simulink model "proceso_simulacion_1"  (Simulink 7.5)
settings: Solver=ode3  StartTime=0.0  StopTime=16000  FixedStep=0.5  RelTol=1e-3
libraries: realtime_pacer_lib x1
settings Model: Creator=cliente  LastModifiedBy=Administrador

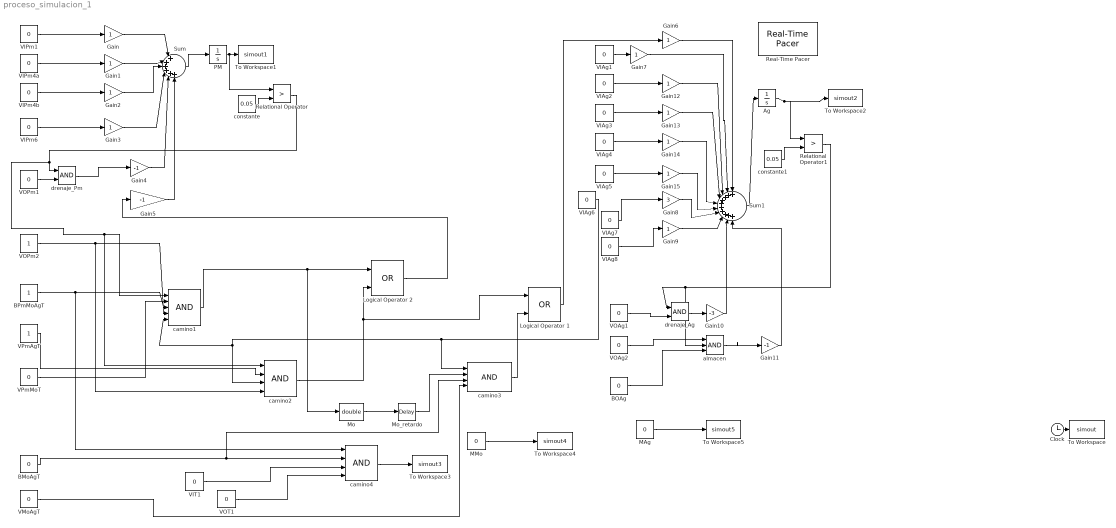
== system proceso_simulacion_1 ==
  Ag : Integrator
  BMoAgT : Constant  Value=0  OutDataType=fixdt(1, 16)  OutScaling=2^0
  BOAg : Constant  Value=0  OutDataType=fixdt(1, 16)  OutScaling=2^0
  BPmMoAgT : Constant  OutDataType=fixdt(1, 16)  OutScaling=2^0
  Clock : Clock
      settings: Decimation=10
  Gain{,1..3,6..7,9,12..15} (11 alike) : Gain  ParameterDataType=fixdt(1, 16)  ParameterScaling=2^0  OutDataType=fixdt(1, 16)  OutScaling=2^0
  Gain10 : Gain  Gain=-3  ParameterDataType=fixdt(1, 16)  ParameterScaling=2^0  OutDataType=fixdt(1, 16)  OutScaling=2^0
  Gain11 : Gain  Gain=-1  ParameterDataType=fixdt(1, 16)  ParameterScaling=2^0  OutDataType=fixdt(1, 16)  OutScaling=2^0
  Gain4 : Gain  Gain=-1  ParameterDataType=fixdt(1, 16)  ParameterScaling=2^0  OutDataType=fixdt(1, 16)  OutScaling=2^0
  Gain5 : Gain  Gain=-1  ParameterDataType=fixdt(1, 16)  ParameterScaling=2^0  OutDataType=fixdt(1, 16)  OutScaling=2^0
  Gain8 : Gain  Gain=3  ParameterDataType=fixdt(1, 16)  ParameterScaling=2^0  OutDataType=fixdt(1, 16)  OutScaling=2^0
  Logical Operator 1 : Logic  Operator=OR  AllPortsSameDT=off  OutDataTypeMode=Specify via dialog  LogicDataType=fixdt(1,16)  OutDataTypeStr=fixdt(1,16)
  Logical Operator 2 : Logic  Operator=OR  AllPortsSameDT=off  OutDataTypeMode=Specify via dialog  LogicDataType=fixdt(1,16)  OutDataTypeStr=fixdt(1,16)
  MAg : Constant  Value=0  OutDataType=fixdt(1, 16)  OutScaling=2^0
  MMo : Constant  Value=0  OutDataType=fixdt(1, 16)  OutScaling=2^0
  Mo : DataTypeConversion  OutDataTypeMode=double  OutDataType=fixdt(1, 16)  OutScaling=2^0  OutDataTypeStr=double
  Mo_retardo : TransportDelay  DelayTime=0.5
  PM : Integrator
  Real-Time Pacer : realtime_pacer_lib/Real-Time Pacer  simTimePerRealTime=1.35
  Relational Operator : RelationalOperator  Operator=>  LogicOutDataTypeMode=boolean  LogicDataType=fixdt(0, 8)  OutDataTypeStr=boolean
  Relational Operator1 : RelationalOperator  Operator=>  LogicOutDataTypeMode=boolean  LogicDataType=fixdt(0, 8)  OutDataTypeStr=boolean
  Sum : Sum  Inputs=|++++++  OutDataType=fixdt(1, 16)  OutScaling=2^0
  Sum1 : Sum  Inputs=++++++++++  OutDataType=fixdt(1, 16)  OutScaling=2^0
  To Workspace : ToWorkspace  VariableName=simout  SampleTime=-1  SaveFormat=Array
  To Workspace1 : ToWorkspace  VariableName=simout1  SampleTime=-1  SaveFormat=Array
  To Workspace2 : ToWorkspace  VariableName=simout2  SampleTime=-1  SaveFormat=Array
  To Workspace3 : ToWorkspace  VariableName=simout3  SampleTime=-1  SaveFormat=Array
  To Workspace4 : ToWorkspace  VariableName=simout4  SampleTime=-1  SaveFormat=Array
  To Workspace5 : ToWorkspace  VariableName=simout5  SampleTime=-1  SaveFormat=Array
  VIAg{1..8} (8 alike) : Constant  Value=0  OutDataType=fixdt(1, 16)  OutScaling=2^0
  VIPm1 : Constant  Value=0  OutDataType=fixdt(1, 16)  OutScaling=2^0
  VIPm4a : Constant  Value=0  OutDataType=fixdt(1, 16)  OutScaling=2^0
  VIPm4b : Constant  Value=0  OutDataType=fixdt(1, 16)  OutScaling=2^0
  VIPm6 : Constant  Value=0  OutDataType=fixdt(1, 16)  OutScaling=2^0
  VIT1 : Constant  Value=0  OutDataType=fixdt(1, 16)  OutScaling=2^0
  VMoAgT : Constant  Value=0  OutDataType=fixdt(1, 16)  OutScaling=2^0
  VOAg1 : Constant  Value=0  OutDataType=fixdt(1, 16)  OutScaling=2^0
  VOAg2 : Constant  Value=0  OutDataType=fixdt(1, 16)  OutScaling=2^0
  VOPm1 : Constant  Value=0  OutDataType=fixdt(1, 16)  OutScaling=2^0
  VOPm2 : Constant  OutDataType=fixdt(1, 16)  OutScaling=2^0
  VOT1 : Constant  Value=0  OutDataType=fixdt(1, 16)  OutScaling=2^0
  VPmAgT : Constant  OutDataType=fixdt(1, 16)  OutScaling=2^0
  VPmMoT : Constant  Value=0  OutDataType=fixdt(1, 16)  OutScaling=2^0
  almacen : Logic  Inputs=3  AllPortsSameDT=off  OutDataTypeMode=Specify via dialog  LogicDataType=fixdt(1,16)  OutDataTypeStr=fixdt(1,16)
  camino1 : Logic  Inputs=5  AllPortsSameDT=off  OutDataTypeMode=Specify via dialog  LogicDataType=fixdt(1,16)  OutDataTypeStr=fixdt(1,16)
  camino2 : Logic  Inputs=4  AllPortsSameDT=off  OutDataTypeMode=Specify via dialog  LogicDataType=fixdt(1,16)  OutDataTypeStr=fixdt(1,16)
  camino3 : Logic  Inputs=4  AllPortsSameDT=off  OutDataTypeMode=boolean  LogicDataType=fixdt(0, 8)  OutDataTypeStr=boolean
  camino4 : Logic  Inputs=4  AllPortsSameDT=off  OutDataTypeMode=Specify via dialog  LogicDataType=fixdt(1,16)  OutDataTypeStr=fixdt(1,16)
  constante : Constant  Value=0.05  OutDataType=fixdt(1, 16)  OutScaling=2^0
  constante1 : Constant  Value=0.05  OutDataType=fixdt(1, 16)  OutScaling=2^0
  drenaje_Ag : Logic  AllPortsSameDT=off  OutDataTypeMode=Specify via dialog  LogicDataType=fixdt(1,16)  OutDataTypeStr=fixdt(1,16)
  drenaje_Pm : Logic  AllPortsSameDT=off  OutDataTypeMode=Specify via dialog  LogicDataType=fixdt(1,16)  OutDataTypeStr=fixdt(1,16)
  wires:
  Gain/1 -> Sum/1
  Gain1/1 -> Sum/2
  Gain2/1 -> Sum/3
  VIPm4b/1 -> Gain2/1
  VIPm4a/1 -> Gain1/1
  VIPm1/1 -> Gain/1
  Sum/1 -> PM/1
  VIPm6/1 -> Gain3/1
  Gain3/1 -> Sum/4
  Gain4/1 -> Sum/5
  Gain5/1 -> Sum/6
  PM/1 -> To Workspace1/1, Relational Operator/1
  Clock/1 -> To Workspace/1
  constante/1 -> Relational Operator/2
  Relational Operator/1 -> drenaje_Pm/1, camino1/1, camino2/1
  VOPm1/1 -> drenaje_Pm/2
  drenaje_Pm/1 -> Gain4/1
  VPmMoT/1 -> camino1/2
  VMoAgT/1 -> camino3/4
  BPmMoAgT/1 -> camino4/1, camino1/3
  BMoAgT/1 -> camino4/2, camino3/3
  camino1/1 -> Logical Operator 2/1, Mo/1
  camino2/1 -> Logical Operator 2/2, Logical Operator 1/1
  Logical Operator 2/1 -> Gain5/1
  VIAg1/1 -> Gain7/1
  VIAg7/1 -> Gain8/1
  VIAg8/1 -> Gain9/1
  Gain6/1 -> Sum1/1
  Gain7/1 -> Sum1/2
  Sum1/1 -> Ag/1
  constante1/1 -> Relational Operator1/2
  Relational Operator1/1 -> drenaje_Ag/1, almacen/2
  VOAg1/1 -> drenaje_Ag/2
  drenaje_Ag/1 -> Gain10/1
  VOAg2/1 -> almacen/1
  BOAg/1 -> almacen/3
  almacen/1 -> Gain11/1
  VIT1/1 -> camino4/3
  VOT1/1 -> camino4/4
  camino4/1 -> To Workspace3/1
  MMo/1 -> To Workspace4/1
  MAg/1 -> To Workspace5/1
  VPmAgT/1 -> camino2/2
  Logical Operator 1/1 -> Gain6/1
  Mo/1 -> Mo_retardo/1
  VOPm2/1 -> camino2/4, camino1/4
  VIAg2/1 -> Gain12/1
  VIAg3/1 -> Gain13/1
  VIAg4/1 -> Gain14/1
  VIAg5/1 -> Gain15/1
  Gain12/1 -> Sum1/3
  Gain13/1 -> Sum1/4
  Gain14/1 -> Sum1/5
  Gain15/1 -> Sum1/6
  Gain8/1 -> Sum1/7
  Gain9/1 -> Sum1/8
  Gain10/1 -> Sum1/9
  Gain11/1 -> Sum1/10
  Ag/1 -> To Workspace2/1, Relational Operator1/1
  Mo_retardo/1 -> camino3/2
  camino3/1 -> Logical Operator 1/2
  VIAg6/1 -> camino3/1, camino2/3, camino1/5
